simulink library "megacorefunctions_alteradspbuilder2"  (Simulink 7.6)
settings: Solver=ode45  StartTime=0.0  StopTime=10.0  RelTol=1e-3
InitFcn:
  | %% DSPBuilder Start
  | alt_dspbuilder_update_model(bdroot)
  | %% DSPBuilder End
undefined symbols (not defined in the file): alt_dspbuilder_internal_init_blackbox_flow, alt_dspbuilder_load_block, alt_dspbuilder_update_external_RAM
libraries: alt_dspbuilder_internal_BusSink x5, alt_dspbuilder_internal_BusSource x3, allblocks_alteradspbuilder2 x2, alt_dspbuilder_internal_Entity x1
settings Model: Creator=swbuild  LastModifiedBy=swbuild

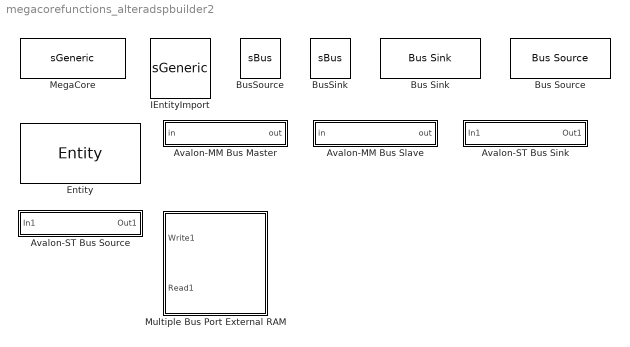
== system megacorefunctions_alteradspbuilder2 ==
  Avalon-MM Bus Master : Subsystem  mask(Avalon-MM Bus Master AlteraBlockset){iofile=D:\\megacorefunctions%5Falteradspbuilder2_Avalon-MM+Bus+Master_waitrequest.salt,D:\\megacorefunctions%5Falteradspbuilder2_Avalon-MM+Bus+Master_address.capture,D:\\megacorefunctions%5Falteradspbuilder2_Avalon-MM+Bus+Master_read.capture,D:\\megacorefunctions%5Falteradspbuilder2_Avalon-MM+Bus+Master_readdata.salt,, SpecifyClock=off, clock=, addrWidth=2, addrType=Read, BusType=Signed Integer, bwl=8, bwr=0, byteEnable=off, flowCtrl=off, pipeline=off, flush=off, burst=off, maxBurst=4, irq=off, irq_mode=Prioritized, externalType=Inferred, PORTTYPE=Input, internalbustype=AVALON_MM, externalbustype=Memory, root=allblocks_alteradspbuilder2/Avalon-MM Master}
      mask prompts: SpecifyClock "Specify Clock"; addrWidth "Address Width"; addrType "Address Type"; BusType "DataType"; bwl "[number of bits].[]"; bwr "[].[number of bits]"; byteEnable "Allow Byte Enable"; flowCtrl "Allow Flow Control"; pipeline "Allow Pipeline Transfers"; flush "Use Flush Signal"; burst "Allow Burst Transfers"; maxBurst "Maximum Burst Size"; irq "Receive IRQ"; irq_mode "IRQ Mode"; externalType "External Type"; PORTTYPE "TYPE"
      mask help: Defines a collection of ports for connection to an SOPC Builder system when your design functions as an Avalon Memory-Mapped master interface.
      mask init:
      | alt_dspbuilder_internal_initBusPortBlock('BlockFactory', 'com.altera.dspbuilder.blockset.avalonmm.BusMaster', { iofile get_param(gcb, 'SpecifyClock') clock addrWidth get_param(gcb, 'addrType') get_param(gcb, 'BusType') bwl bwr byteEnable get_param(gcb, 'flowCtrl') get_param(gcb, 'pipeline') get_param(gcb, 'flush') get_param(gcb, 'burst') maxBurst get_param(gcb, 'irq') get_param(gcb, 'irq_mode') externalType PORTTYPE internalbustype externalbustype root });
      mask Help: helpview(char(com.altera.dspbuilder.simulation.Cache.getBlockTemplate('BlockFactory', 'com.altera.dspbuilder.blockset.avalonmm.BusMaster').getHelpFile))
      mask StyleString: edit,checkbox,edit,edit,popup(Read|Write|Read/Write),popup(Signed Integer|Unsigned Integer|Signed Fractional|Unsigned Fractional),edit,edit,checkbox,checkbox,checkbox,checkbox,checkbox,edit,checkbox,popup(Prioritized|Indiviual Signals),popup(Inferred|Simulink Fixed Point Type|Double),edit,edit,edit,edit
      mask CallbackString: |alt_dspbuilder_update_gui('BlockFactory', 'com.altera.dspbuilder.blockset.avalonmm.BusMaster', 'SpecifyClock', 1);|||alt_dspbuilder_update_gui('BlockFactory', 'com.altera.dspbuilder.blockset.avalonmm.BusMaster', 'addrType', 4);|alt_dspbuilder_update_gui('BlockFactory', 'com.altera.dspbuilder.blockset.avalonmm.BusMaster', 'BusType', 5);||||alt_dspbuilder_update_gui('BlockFactory', 'com.altera.dspbuilder.blockset.avalonmm.BusMaster', 'flowCtrl', 9);|alt_dspbuilder_update_gui('BlockFactory', 'com.altera.dspbuilder.blockset.avalonmm.BusMaster', 'pipeline', 10);|alt_dspbuilder_update_gui('BlockFactory', 'com.altera.dspbuilder.blockset.avalonmm.BusMaster', 'flush', 11);|alt_dspbuilder_update_gui('BlockFactory', 'com.altera.dspbuilder.blockset.avalonmm.BusMaster', 'burst', 12);||alt_dspbuilder_update_gui('BlockFactory', 'com.altera.dspbuilder.blockset.avalonmm.BusMaster', 'irq', 14);|alt_dspbuilder_update_gui('BlockFactory', 'com.altera.dspbuilder.blockset.avalonmm.BusMaster', 'irq_mode', 15);|||||
      mask Display: plot([-25 19 29 19 -25 -25]*-1, [0 0 -10 -20 -20 0] - 0);plot([11 21 11]*-1, [0 -10 -20] - 0);plot([15 25 15]*-1, [0 -10 -20] - 0);text(-5*-1, -10, 'AV-MM Master', 'horizontalAlignment','center','verticalAlignment','middle');
  Avalon-MM Bus Slave : Subsystem  mask(Avalon-MM Bus Slave AlteraBlockset){iofile=D:\\megacorefunctions%5Falteradspbuilder2_Avalon-MM+Bus+Slave_address.salt,D:\\megacorefunctions%5Falteradspbuilder2_Avalon-MM+Bus+Slave_write.salt,D:\\megacorefunctions%5Falteradspbuilder2_Avalon-MM+Bus+Slave_writedata.salt,D:\\megacorefunctions%5Falteradspbuilder2_Avalon-MM+Bus+Slave_byteenable.salt,, SpecifyClock=off, clock=, addrWidth=2, addrAlignment=Dynamic, addrType=Write, BusType=Unsigned Integer, bwl=16, bwr=0, byteEnable=on, flowCtrl=off, pipeline=off, waitStateFormat=Fixed, readWaitStateCycles=0, writeWaitStateCycles=0, readLatencyFormat=Fixed, readLatencyCycles=0, burst=off, maxBurst=4, irq=off, receiveBeginTransfer=off, useChipSelect=off, externalType=Inferred, PORTTYPE=Output, internalbustype=AVALON_MM, externalbustype=Memory, root=allblocks_alteradspbuilder2/Avalon-MM Slave}
      mask prompts: SpecifyClock "Specify Clock"; addrWidth "Address Width"; addrAlignment "Address Alignment"; addrType "Address Type"; BusType "DataType"; bwl "[number of bits].[]"; bwr "[].[number of bits]"; byteEnable "Allow Byte Enable"; flowCtrl "Allow Flow Control"; pipeline "Allow Pipeline Transfers"; waitStateFormat "Wait-State Format"; readWaitStateCycles "Read Wait-State Cycles"; writeWaitStateCycles "Write Wait-State Cycles"; readLatencyFormat "Read Latency Format"; readLatencyCycles "Read Latency Cycles"; burst "Allow Burst Transfers"; maxBurst "Maximum Burst Size"; irq "Output IRQ"; receiveBeginTransfer "Receive BeginTransfer"; useChipSelect "Use Chip Select"; externalType "External Type"; PORTTYPE "TYPE"
      mask help: Defines a collection of ports for connection to an SOPC Builder system when your design functions as an Avalon Memory-Mapped slave interface.
      mask init:
      | alt_dspbuilder_internal_initBusPortBlock('BlockFactory', 'com.altera.dspbuilder.blockset.avalonmm.BusSlave', { iofile get_param(gcb, 'SpecifyClock') clock addrWidth addrAlignment get_param(gcb, 'addrType') get_param(gcb, 'BusType') bwl bwr byteEnable flowCtrl pipeline get_param(gcb, 'waitStateFormat') readWaitStateCycles writeWaitStateCycles readLatencyFormat readLatencyCycles get_param(gcb, 'burst') maxBurst irq receiveBeginTransfer useChipSelect externalType PORTTYPE internalbustype externalbustype root });
      mask Help: helpview(char(com.altera.dspbuilder.simulation.Cache.getBlockTemplate('BlockFactory', 'com.altera.dspbuilder.blockset.avalonmm.BusSlave').getHelpFile))
      mask StyleString: edit,checkbox,edit,edit,popup(Dynamic|Native),popup(Read|Write|Read/Write),popup(Signed Integer|Unsigned Integer|Signed Fractional|Unsigned Fractional),edit,edit,checkbox,checkbox,checkbox,popup(Fixed|Variable),edit,edit,popup(Fixed|Variable),edit,checkbox,edit,checkbox,checkbox,checkbox,popup(Inferred|Simulink Fixed Point Type|Double),edit,edit,edit,edit
      mask CallbackString: |alt_dspbuilder_update_gui('BlockFactory', 'com.altera.dspbuilder.blockset.avalonmm.BusSlave', 'SpecifyClock', 1);||||alt_dspbuilder_update_gui('BlockFactory', 'com.altera.dspbuilder.blockset.avalonmm.BusSlave', 'addrType', 5);|alt_dspbuilder_update_gui('BlockFactory', 'com.altera.dspbuilder.blockset.avalonmm.BusSlave', 'BusType', 6);||||||alt_dspbuilder_update_gui('BlockFactory', 'com.altera.dspbuilder.blockset.avalonmm.BusSlave', 'waitStateFormat', 12);|||||alt_dspbuilder_update_gui('BlockFactory', 'com.altera.dspbuilder.blockset.avalonmm.BusSlave', 'burst', 17);|||||||||
      mask Display: plot([-25 19 29 19 -25 -25]*1, [0 0 -10 -20 -20 0] - 0);plot([11 21 11]*1, [0 -10 -20] - 0);plot([15 25 15]*1, [0 -10 -20] - 0);text(-5*1, -10, 'AV-MM Slave', 'horizontalAlignment','center','verticalAlignment','middle');
  Avalon-ST Bus Sink : Subsystem  mask(Avalon-ST Bus Sink AlteraBlockset){iofile=, SpecifyClock=off, clock=, BusType=Unsigned Integer, bwl=8, bwr=0, symbolWidth=8, symbolsPerBeat=0, endOfPacket=off, startOfPacket=off, readyLatency=1, externalType=Inferred, PORTTYPE=Output, internalbustype=AVALON_ST, externalbustype=Stream, root=allblocks_alteradspbuilder2/Avalon-ST Sink}
      mask prompts: SpecifyClock "Specify Clock"; BusType "DataType"; bwl "[number of bits].[]"; bwr "[].[number of bits]"; symbolWidth "Symbol Width"; endOfPacket "Use endofpacket"; startOfPacket "Use startofpacket"; readyLatency "Ready Latency"; externalType "External Type"; PORTTYPE "TYPE"
      mask help: Defines a collection of ports for connection to an SOPC Builder system when your design functions as an Avalon-ST source.
      mask init:
      | alt_dspbuilder_internal_initBusPortBlock('BlockFactory', 'com.altera.dspbuilder.blockset.avalonst.BusSink', { iofile get_param(gcb, 'SpecifyClock') clock get_param(gcb, 'BusType') bwl bwr symbolWidth symbolsPerBeat get_param(gcb, 'endOfPacket') get_param(gcb, 'startOfPacket') readyLatency externalType PORTTYPE internalbustype externalbustype root });
      mask Help: helpview(char(com.altera.dspbuilder.simulation.Cache.getBlockTemplate('BlockFactory', 'com.altera.dspbuilder.blockset.avalonst.BusSink').getHelpFile))
      mask StyleString: edit,checkbox,edit,popup(Signed Integer|Unsigned Integer|Signed Fractional|Unsigned Fractional),edit,edit,edit,edit,checkbox,checkbox,edit,popup(Inferred|Simulink Fixed Point Type|Double),edit,edit,edit,edit
      mask CallbackString: |alt_dspbuilder_update_gui('BlockFactory', 'com.altera.dspbuilder.blockset.avalonst.BusSink', 'SpecifyClock', 1);||alt_dspbuilder_update_gui('BlockFactory', 'com.altera.dspbuilder.blockset.avalonst.BusSink', 'BusType', 3);|||||alt_dspbuilder_update_gui('BlockFactory', 'com.altera.dspbuilder.blockset.avalonst.BusSink', 'endOfPacket', 8);|alt_dspbuilder_update_gui('BlockFactory', 'com.altera.dspbuilder.blockset.avalonst.BusSink', 'startOfPacket', 9);||||||
  Avalon-ST Bus Source : Subsystem  mask(Avalon-ST Bus Source AlteraBlockset){iofile=, SpecifyClock=off, clock=, BusType=Unsigned Integer, bwl=8, bwr=0, symbolWidth=8, symbolsPerBeat=0, endOfPacket=off, startOfPacket=off, readyLatency=1, externalType=Inferred, PORTTYPE=Input, internalbustype=AVALON_ST, externalbustype=Stream, root=allblocks_alteradspbuilder2/Avalon-ST Source}
      mask prompts: SpecifyClock "Specify Clock"; BusType "DataType"; bwl "[number of bits].[]"; bwr "[].[number of bits]"; symbolWidth "Symbol Width"; endOfPacket "Use endofpacket"; startOfPacket "Use startofpacket"; readyLatency "Ready Latency"; externalType "External Type"; PORTTYPE "TYPE"
      mask help: Defines a collection of ports for connection to an SOPC Builder system when your design functions as an Avalon-ST source.
      mask init:
      | alt_dspbuilder_internal_initBusPortBlock('BlockFactory', 'com.altera.dspbuilder.blockset.avalonst.BusSource', { iofile get_param(gcb, 'SpecifyClock') clock get_param(gcb, 'BusType') bwl bwr symbolWidth symbolsPerBeat get_param(gcb, 'endOfPacket') get_param(gcb, 'startOfPacket') readyLatency externalType PORTTYPE internalbustype externalbustype root });
      mask Help: helpview(char(com.altera.dspbuilder.simulation.Cache.getBlockTemplate('BlockFactory', 'com.altera.dspbuilder.blockset.avalonst.BusSource').getHelpFile))
      mask StyleString: edit,checkbox,edit,popup(Signed Integer|Unsigned Integer|Signed Fractional|Unsigned Fractional),edit,edit,edit,edit,checkbox,checkbox,edit,popup(Inferred|Simulink Fixed Point Type|Double),edit,edit,edit,edit
      mask CallbackString: |alt_dspbuilder_update_gui('BlockFactory', 'com.altera.dspbuilder.blockset.avalonst.BusSource', 'SpecifyClock', 1);||alt_dspbuilder_update_gui('BlockFactory', 'com.altera.dspbuilder.blockset.avalonst.BusSource', 'BusType', 3);|||||alt_dspbuilder_update_gui('BlockFactory', 'com.altera.dspbuilder.blockset.avalonst.BusSource', 'endOfPacket', 8);|alt_dspbuilder_update_gui('BlockFactory', 'com.altera.dspbuilder.blockset.avalonst.BusSource', 'startOfPacket', 9);||||||
  Bus Sink : alt_dspbuilder_internal_BusSink/Bus Sink  SystemSampleTime=-1  sources=0  sinks=0
  Bus Source : alt_dspbuilder_internal_BusSource/Bus Source  SystemSampleTime=-1  sources=0  sinks=0
  BusSink : S-Function  LoadFcn=alt_dspbuilder_load_block(gcb, 'BlockFactory', 'com.altera.dspbuilder.blockset.buses.BusSink');  FunctionName=sBus  Parameters=busType sources sinks  EnableBusSupport=off  mask(Bus Wire Sink AlteraBlockset){busType=AVALON_ST, sources=, sinks=}
      mask prompts: busType "Bus Type"; sinks "Sources"
      mask init:
      | alt_dspbuilder_init('BlockFactory', 'com.altera.dspbuilder.blockset.buses.BusSink', { busType sources sinks });
      settings: CopyFcn=alt_dspbuilder_add_block(gcb, 'BlockFactory', 'com.altera.dspbuilder.blockset.buses.BusSink');  DeleteFcn=com.altera.dspbuilder.simulation.Mask.delete(gcb);  UndoDeleteFcn=alt_dspbuilder_add_block(gcb, 'BlockFactory', 'com.altera.dspbuilder.blockset.buses.BusSink');  PostSaveFcn=alt_dspbuilder_block_saved(gcb);  NameChangeFcn=alt_dspbuilder_block_renamed(gcb);
      mask Help: helpview(char(com.altera.dspbuilder.simulation.Cache.getBlockTemplate('BlockFactory', 'com.altera.dspbuilder.blockset.buses.BusSink').getHelpFile))
      mask Display:
      | port_label('input', 1, '<');
      | disp(busType)
  BusSource : S-Function  LoadFcn=alt_dspbuilder_load_block(gcb, 'BlockFactory', 'com.altera.dspbuilder.blockset.buses.BusSource');  FunctionName=sBus  Parameters=busType sources sinks  EnableBusSupport=off  mask(Bus Wire Source AlteraBlockset){busType=AVALON_ST, sources=, sinks=}
      mask prompts: busType "Bus Type"; sinks "Sources"
      mask init:
      | alt_dspbuilder_init('BlockFactory', 'com.altera.dspbuilder.blockset.buses.BusSource', { busType sources sinks });
      settings: CopyFcn=alt_dspbuilder_add_block(gcb, 'BlockFactory', 'com.altera.dspbuilder.blockset.buses.BusSource');  DeleteFcn=com.altera.dspbuilder.simulation.Mask.delete(gcb);  UndoDeleteFcn=alt_dspbuilder_add_block(gcb, 'BlockFactory', 'com.altera.dspbuilder.blockset.buses.BusSource');  PostSaveFcn=alt_dspbuilder_block_saved(gcb);  NameChangeFcn=alt_dspbuilder_block_renamed(gcb);
      mask Help: helpview(char(com.altera.dspbuilder.simulation.Cache.getBlockTemplate('BlockFactory', 'com.altera.dspbuilder.blockset.buses.BusSource').getHelpFile))
      mask Display:
      | port_label('output', 1, '>');
      | disp(busType)
  Entity : alt_dspbuilder_internal_Entity/Entity  SystemSampleTime=-1  entityDisplayName=Entity  showResets=off  n_input_port=0  n_output_port=0  busNames=0  busTypes=0  busDirections=0  busInputRoles=0  busOutputRoles=0
  IEntityImport : S-Function  LoadFcn=alt_dspbuilder_load_block(gcb, 'BlockFactory', 'com.altera.dspbuilder.blockset.altlab.IEntityImport');  FunctionName=sGeneric  Parameters=entityName entityVersion searchPath entityDisplayName entityParameterMap showResets n_input_port n_output_port inNames inBwls inBwrs inTypes inDelayed outNames outBwls outBwrs outTypes array_clocks resetNames resetTypes resetLengths allowFloatingPointOverride busNames busTypes busDirections busInputRoles busOutputRoles  EnableBusSupport=off  mask(IEntityImport AlteraBlockset){entityName=, entityVersion=, searchPath=, entityDisplayName=, entityParameterMap=, showResets=off, n_input_port=0, n_output_port=0, inNames=, inBwls=, inBwrs=, inTypes=, inDelayed=, outNames=, outBwls=, outBwrs=, outTypes=, array_clocks=, resetNames=, resetTypes=, resetLengths=, allowFloatingPointOverride=off, busNames=, busTypes=, busDirections=, busInputRoles=, busOutputRoles=}
      mask prompts: entityName "IEntity Name"; entityVersion "IEntity Version"; searchPath "IEntity Search Path"; entityDisplayName "IEntity Display Name"; entityParameterMap "IEntity Parameterization"; showResets "Show reset ports"; inNames "Input Port Names"; inBwls "Input Bitwidth Lefts"; inBwrs "Input Bitwidth Rights"; inTypes "Input Types"; inDelayed "Input Delayed Flags"; outNames "Output Port Names"; outBwls "Output Bitwidth Lefts"; outBwrs "Output Bitwidth Rights"; outTypes "Output Types"; array_clocks "Clocks"; resetNames "Reset Names"; resetTypes "Reset Types"; resetLengths "Reset Lengths"; busNames "Bus Names"; busTypes "Bus Types"; busDirections "Bus Directions"; busInputRoles "Bus Input Roles"; busOutputRoles "Bus Output Roles"
      mask init:
      | alt_dspbuilder_init('BlockFactory', 'com.altera.dspbuilder.blockset.altlab.IEntityImport', { entityName entityVersion searchPath entityDisplayName entityParameterMap showResets n_input_port n_output_port inNames inBwls inBwrs inTypes inDelayed outNames outBwls outBwrs outTypes array_clocks resetNames resetTypes resetLengths allowFloatingPointOverride busNames busTypes busDirections busInputRoles busOutputRoles });
      settings: CopyFcn=alt_dspbuilder_add_block(gcb, 'BlockFactory', 'com.altera.dspbuilder.blockset.altlab.IEntityImport');  DeleteFcn=com.altera.dspbuilder.simulation.Mask.delete(gcb);  UndoDeleteFcn=alt_dspbuilder_add_block(gcb, 'BlockFactory', 'com.altera.dspbuilder.blockset.altlab.IEntityImport');  PostSaveFcn=alt_dspbuilder_block_saved(gcb);  NameChangeFcn=alt_dspbuilder_block_renamed(gcb);
      settings: OpenFcn=|
      | com.altera.dspbuilder.simulation.Mask.simpleInit('BlockFactory', 'com.altera.dspbuilder.blockset.altlab.IEntityImport', bdroot(gcb), gcb);
      | alt_dspbuilder_internal_entityConfiguration(gcb)
      mask Help: helpview(char(com.altera.dspbuilder.simulation.Cache.getBlockTemplate('BlockFactory', 'com.altera.dspbuilder.blockset.altlab.IEntityImport').getHelpFile))
      mask Display: disp(entityDisplayName);
  MegaCore : S-Function  LoadFcn=alt_dspbuilder_load_block(gcb, 'BlockFactory', 'com.altera.dspbuilder.blockset.megacorefunctions.MegaCore');  InitFcn=alt_dspbuilder_internal_init_blackbox_flow;  FunctionName=sGeneric  Parameters=entityName inNames inBwls inBwrs inTypes inDelayed outNames outBwls outBwrs outTypes xmlmapfile launch_params is_megacore use_dynamic_feedthrough_data use_alphabetical_port_ordering vofile n_input_port n_output_port core_dir core_name clockname flow_dir core_version NewVariation VhdlVariationDate VhdlVariationName systemC_model_file use_systemC_model wizard resetNames resetTypes resetLengths inptype outptype allowFloatingPointOverride  EnableBusSupport=off  mask(MegaCore AlteraBlockset){entityName=, inNames=, inBwls=, inBwrs=, inTypes=, inDelayed=, outNames=, outBwls=, outBwrs=, outTypes=, xmlmapfile=SimgenCMap.xml, launch_params=, is_megacore=on, use_dynamic_feedthrough_data=on, use_alphabetical_port_ordering=on, vofile=test_core.vo, n_input_port=0, n_output_port=0, core_dir=C:\\altera\\71\\ip\\fft\\lib\\ip_toolbench, core_name=, clockname=, flow_dir=C:\\altera\\71\\ip\\fft\\lib\\..\\..\\common\\ip_toolbench\\v1.3.0\\bin, core_version=, NewVariation=on, VhdlVariationDate=09-Nov-2006 14:30:07, VhdlVariationName=test_core.vhd, systemC_model_file=, use_systemC_model=off, wizard=fft, resetNames=, resetTypes=, resetLengths=, inptype=, outptype=, allowFloatingPointOverride=off}
      mask prompts: entityName "Entity Name"; inNames "Input port names"; inBwls "Input Bitwidth lefts"; inBwrs "Input Bitwidth rights"; inTypes "Input Types"; inDelayed "Input Delayed Flags"; outNames "Output port names"; outBwls "Output Bitwidth lefts"; outBwrs "Output Bitwidth rights"; outTypes "Output Types"; systemC_model_file "SystemC model file"; use_systemC_model "Use SystemC bit-accurate model"; resetNames "array_clocks"; resetTypes "array_clocks"; resetLengths "array_clocks"
      mask help: When you double-click on this block, it opens the MegaCore function user interface which allows you to generate all the files required to integrate a parameterized MegaCore function variation into the model.
      mask init:
      | alt_dspbuilder_init('BlockFactory', 'com.altera.dspbuilder.blockset.megacorefunctions.MegaCore', { entityName inNames inBwls inBwrs inTypes inDelayed outNames outBwls outBwrs outTypes xmlmapfile launch_params is_megacore use_dynamic_feedthrough_data use_alphabetical_port_ordering vofile n_input_port n_output_port core_dir core_name clockname flow_dir core_version NewVariation VhdlVariationDate VhdlVariationName systemC_model_file use_systemC_model wizard resetNames resetTypes resetLengths inptype outptype allowFloatingPointOverride });
      settings: DeleteFcn=com.altera.dspbuilder.simulation.Mask.delete(gcb);  UndoDeleteFcn=alt_dspbuilder_add_block(gcb, 'BlockFactory', 'com.altera.dspbuilder.blockset.megacorefunctions.MegaCore');  PostSaveFcn=alt_dspbuilder_block_saved(gcb);
      settings: CopyFcn=|
      | alt_dspbuilder_add_block(gcb, 'BlockFactory', 'com.altera.dspbuilder.blockset.megacorefunctions.MegaCore');
      | alt_dspbuilder_internal_megacorealtr_copy(gcb)
      settings: NameChangeFcn=|
      | alt_dspbuilder_block_renamed(gcb);
      | alt_dspbuilder_internal_megacorealtr_rename(gcb)
      settings: OpenFcn=|
      | com.altera.dspbuilder.simulation.Mask.simpleInit('BlockFactory', 'com.altera.dspbuilder.blockset.megacorefunctions.MegaCore', bdroot(gcb), gcb);
      | alt_dspbuilder_megacorealtr_launch(gcb, 0, 0)
      mask Help: helpview(char(com.altera.dspbuilder.simulation.Cache.getBlockTemplate('BlockFactory', 'com.altera.dspbuilder.blockset.megacorefunctions.MegaCore').getHelpFile))
      mask Display: disp(' ');
  Multiple Bus Port External RAM : Subsystem  mask{WRITE_INTERFACES=1, READ_INTERFACES=1, DATA_WIDTH=32, ADDRESS_WIDTH=8, WAIT_STATES_PER_WRITE=0, MAXIMUM_LATENCY=1, SIZE=100, OFFSET=0}
      mask prompts: WRITE_INTERFACES "Number of Write Buses"; READ_INTERFACES "Number of Read Buses"; DATA_WIDTH "Data Width"; ADDRESS_WIDTH "Address Width"; WAIT_STATES_PER_WRITE "Wait States Per Write"; MAXIMUM_LATENCY "Maximum Latency"
      mask help:
      | This is a simulation model of an external RAM block.  It can be used to store and retrieve data from a range of addresses.  It is designed specifically to work with the DSP Builder Video and Image Processing blocks, but may be used for other purposes.
      |
      | As it is a simulation only block, it will not generate HDL when SignalCompiler is run.
      |
      | Parameters
      | =========
      | Data Width - the number of bits used for the data (8,16, 32, 64 or 128 bits only)
      | Address Width - number of bits used for the address (between 1 and 32)
      | Wait States Per Write - choose a fixed number of wait states for each write transfer (between 0 to 10)
      | Maximum Latency - set the latency for pipelined read transfer (between 1 and 255)
      | Size, Offset - to use a range of addresses, choose an offset (start address) and size (number of addresses).  The size added to the offset must be less than 2 ^ address width).
      |
      | Note : If 64 or 128 bits are selected for the data width, the block will attempt to register a Simulink fixed point type of the corresponding width.  This will only work if a valid fixed point license is present on the user's machine.  Please refer to the Simulink help for more information about fixed point licenses.
      mask init:
      | system = gcb;
      | paramNames = get_param(system, 'MaskNames');
      | paramsAndCommas = strcat(paramNames,',');
      | paramValues = eval(['{' paramsAndCommas{:} '}'])';
      | alt_dspbuilder_internal_initMultipleBusPortExternalRAM(system,...
      |             WRITE_INTERFACES, READ_INTERFACES, paramNames, paramValues);
      mask Help: helpview(fullfile(alt_dspbuilder_get_quartus_rootdir, 'dsp_builder', 'docs', 'MultiplePortExternalRAM.html'))

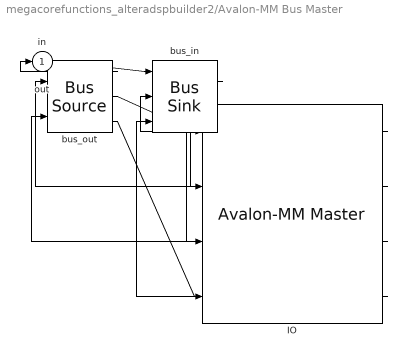
== system megacorefunctions_alteradspbuilder2/Avalon-MM Bus Master ==
  in : Inport
  IO : allblocks_alteradspbuilder2/Avalon-MM Master  SystemSampleTime=-1  iofile=D:\megacorefunctions%5Falteradspbuilder2_Avalon-MM+Bus+Master_IO_waitrequest.salt,D:\megacorefunctions%5Falteradspbuilder2_Avalon-MM+Bus+Master_IO_address.capture,D:\megacorefunctions%5Falteradspbuilder2_Avalon-MM+Bus+Master_IO_read.capture,D:\megacorefunctions%5Falteradspbuilder2_Avalon-MM+Bus+Master_IO_readdata.salt,  SpecifyClock=off  addrWidth=2  addrType=Read  BusType=Signed Integer  bwl=8  bwr=0  byteEnable=off  flowCtrl=off  pipeline=off  flush=off  burst=off  maxBurst=4  irq=off  irq_mode=Prioritized  externalType=Inferred  PORTTYPE=Input
  bus_in : alt_dspbuilder_internal_BusSink/Bus Sink  SystemSampleTime=-1  sources={ 'waitrequest','readdata', }  sinks={ 'address','read', }  busType=AVALON_MM
  bus_out : alt_dspbuilder_internal_BusSource/Bus Source  SystemSampleTime=-1  sources={ 'address','read', }  sinks={ 'waitrequest','readdata', }  busType=Memory
  out : Outport
  wires:
  in/1 -> bus_in/1
  bus_out/1 -> out/1
  bus_out/2 -> IO/1
  IO/1 -> bus_in/2
  bus_in/1 -> IO/2
  IO/2 -> bus_out/1
  bus_in/2 -> IO/3
  IO/3 -> bus_out/2
  bus_out/3 -> IO/4
  IO/4 -> bus_in/3

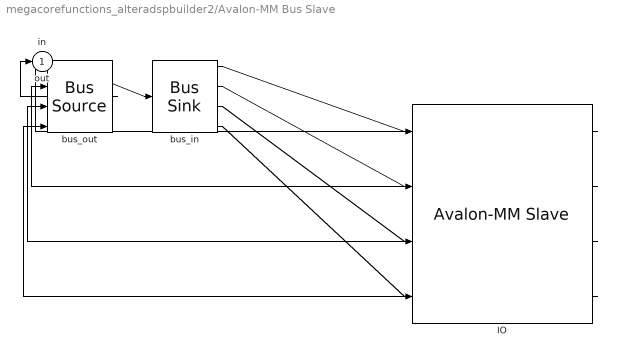
== system megacorefunctions_alteradspbuilder2/Avalon-MM Bus Slave ==
  in : Inport
  IO : allblocks_alteradspbuilder2/Avalon-MM Slave  SystemSampleTime=-1  iofile=D:\megacorefunctions%5Falteradspbuilder2_Avalon-MM+Bus+Slave_IO_address.salt,D:\megacorefunctions%5Falteradspbuilder2_Avalon-MM+Bus+Slave_IO_write.salt,D:\megacorefunctions%5Falteradspbuilder2_Avalon-MM+Bus+Slave_IO_writedata.salt,D:\megacorefunctions%5Falteradspbuilder2_Avalon-MM+Bus+Slave_IO_byteenable.salt,  SpecifyClock=off  addrWidth=2  addrAlignment=Dynamic  addrType=Write  BusType=Unsigned Integer  bwl=16  bwr=0  byteEnable=on  flowCtrl=off  pipeline=off  waitStateFormat=Fixed  readWaitStateCycles=0  writeWaitStateCycles=0  readLatencyFormat=Fixed  readLatencyCycles=0  burst=off  maxBurst=4  irq=off  receiveBeginTransfer=off  useChipSelect=off  externalType=Inferred  PORTTYPE=Output
  bus_in : alt_dspbuilder_internal_BusSink/Bus Sink  SystemSampleTime=-1  sources={ }  sinks={ 'address','write','writedata','byteenable', }  busType=Memory
  bus_out : alt_dspbuilder_internal_BusSource/Bus Source  SystemSampleTime=-1  sources={ 'address','write','writedata','byteenable', }  sinks={ }  busType=AVALON_MM
  out : Outport
  wires:
  in/1 -> bus_in/1
  bus_out/1 -> out/1
  bus_in/1 -> IO/1
  IO/1 -> bus_out/1
  bus_in/2 -> IO/2
  IO/2 -> bus_out/2
  bus_in/3 -> IO/3
  IO/3 -> bus_out/3
  bus_in/4 -> IO/4
  IO/4 -> bus_out/4

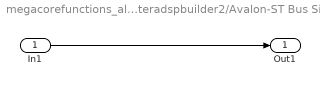
== system megacorefunctions_alteradspbuilder2/Avalon-ST Bus Sink ==
  In1 : Inport
  Out1 : Outport
  wires:
  In1/1 -> Out1/1

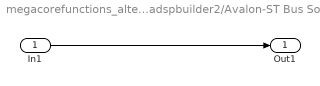
== system megacorefunctions_alteradspbuilder2/Avalon-ST Bus Source ==
  In1 : Inport
  Out1 : Outport
  wires:
  In1/1 -> Out1/1

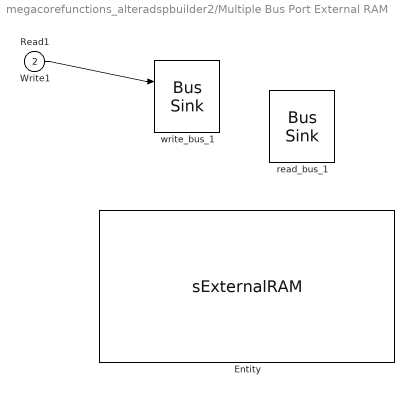
== system megacorefunctions_alteradspbuilder2/Multiple Bus Port External RAM ==
  Write1 : Inport
  Read1 : Inport  Port=2
  Entity : S-Function  InitFcn=alt_dspbuilder_update_external_RAM();  StartFcn=alt_dspbuilder_internal_externalRAMWarning  FunctionName=sExternalRAM  Parameters=WRITE_INTERFACES READ_INTERFACES DATA_WIDTH ADDRESS_WIDTH WAIT_STATES_PER_WRITE MAXIMUM_LATENCY SIZE OFFSET  EnableBusSupport=off  mask{WRITE_INTERFACES=1, READ_INTERFACES=1, DATA_WIDTH=32, ADDRESS_WIDTH=8, WAIT_STATES_PER_WRITE=0, MAXIMUM_LATENCY=1, SIZE=100, OFFSET=0}
      mask prompts: WRITE_INTERFACES "Number of Write Interfaces"; READ_INTERFACES "Number of Read Interfaces"; DATA_WIDTH "Data Width"; ADDRESS_WIDTH "Address Width"; WAIT_STATES_PER_WRITE "Wait States Per Write"; MAXIMUM_LATENCY "Maximum Latency"
      mask help:
      | This is a simulation model of an external RAM block.  It can be used to store and retrieve data from a range of addresses.  It is designed specifically to work with the DSP Builder Video and Image Processing blocks, but may be used for other purposes.
      |
      | As it is a simulation only block, it will not generate HDL when SignalCompiler is run.
      |
      | Parameters
      | =========
      | Data Width - the number of bits used for the data (8,16, 32, 64 or 128 bits only)
      | Address Width - number of bits used for the address (between 1 and 32)
      | Wait States Per Write - choose a fixed number of wait states for each write transfer (between 0 to 10)
      | Maximum Latency - set the latency for pipelined read transfer (between 1 and 255)
      | Size, Offset - to use a range of addresses, choose an offset (start address) and size (number of addresses).  The size added to the offset must be less than 2 ^ address width).
      |
      | Note : If 64 or 128 bits are selected for the data width, the block will attempt to register a Simulink fixed point type of the corresponding width.  This will only work if a valid fixed point license is present on the user's machine.  Please refer to the Simulink help for more information about fixed point licenses.
      mask Display:
      | port_label('input', 1, 'WriteData1');
      | port_label('input', 2, 'WriteAddress1');
      | port_label('input', 3, 'WriteEnable1');
      | port_label('output', 1, 'WriteWaitRequest1');
      | port_label('input', 4, 'WriteData2');
      | port_label('input', 5, 'WriteAddress2');
      | port_label('input', 6, 'WriteEnable2');
      | port_label('output', 2, 'WriteWaitRequest2');
      | port_label('input', 7, 'WriteData3');
      | port_label('input', 8, 'WriteAddress3');
      | port_label('input', 9, 'WriteEnable3');
      | port_label('output', 3, 'WriteWaitRequest3');
      | port_label('input', 10, 'ReadAddress1');
      | port_label('input', 11, 'ReadEnable1');
      | port_label('output', 4, 'ReadData1');
      | port_label('output', 5, 'ReadDataValid1');
      | port_label('output', 6, 'ReadWaitRequest1');
      | port_label('input', 12, 'ReadAddress2');
      | port_label('input', 13, 'ReadEnable2');
      | port_label('output', 7, 'ReadData2');
      | port_label('output', 8, 'ReadDataValid2');
      | port_label('output', 9, 'ReadWaitRequest2');
  read_bus_1 : alt_dspbuilder_internal_BusSink/Bus Sink  SystemSampleTime=-1  sources={'readdata', 'readdatavalid', 'waitrequest'}  sinks={'address', 'read'}  busType=Memory
  write_bus_1 : alt_dspbuilder_internal_BusSink/Bus Sink  SystemSampleTime=-1  sources={'waitrequest'}  sinks={'writedata','address', 'write'}  busType=Memory
  wires:
  Write1/1 -> write_bus_1/1
